simulink model "inverted_pendulum_2023b"  (R2023b)
settings: Solver=VariableStepAuto  StartTime=0.0  StopTime=double(Tsim)  RelTol=1e-3
InitFcn:
  | x0 = [0.0, 0, pi, 0.2];
  | measurementNoiseVariance = 1e-5 * [1, 1, 1, 1];
  | dt = 1e-3;
  | Tsim = 3;
settings Model: Creator=ka59symi  LastModifiedBy=ka59symi

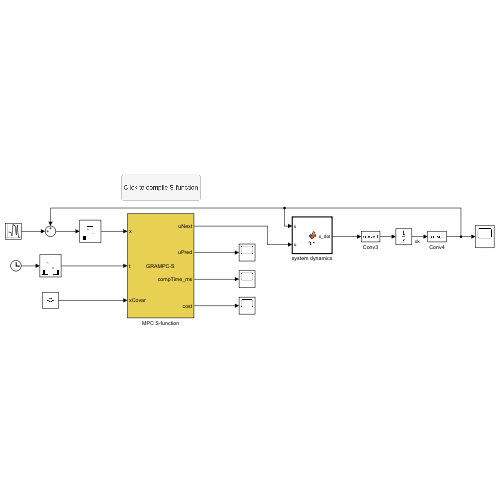
[thumbnail: Simulink's stored preview of the top-level diagram]
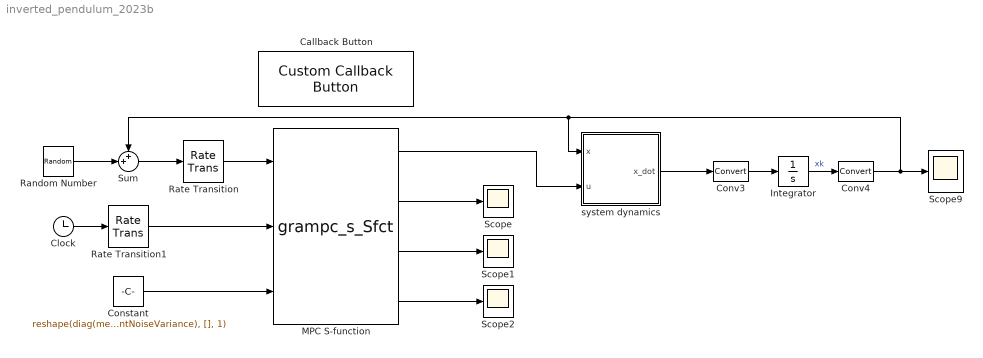
== system inverted_pendulum_2023b ==
  Callback Button : CustomCallbackButton  Configuration="{\"components\":[{\"name\":\"BackgroundImageComponent\",\"settings\":{\"image\":{\"size\":[0,0],\"src\":\"default\",\"srcOrientation\":\"Right\"},\"position\":[0,0,1,1]}},{\"name\":\"ButtonStateComponent\",\"settings\":{\"buttonType\":\"momentary\",\"clickFcn\":\"clc;\\nclear all;\\n\\npath_to_grampc = fileparts(fileparts(cd));\\n\\nprobfct_inc = fullfile(cd, 'inverted_pendulum_problem_description.hpp');\\nprobfct_src = fullfile(cd, 'inverted_pendulum_problem_description.cpp');\\ns_function  = fullfile(cd, 'grampc_s_Sfct.cpp');\\n\\naddpath(fullfile(path_to_grampc, 'matlab'));\\n\\nmake_Sfunction(path_to_grampc, probfct_inc, probfct_src, s_function);\",\"onValue\":1,\"position\":[0,0,1,1],\"pressDelay\":\"500\",\"pressFcn\":\"\",\"repeatInterval\":\"0\",\"states\":[{\"horizontalAlignment\":\"center\",\"image\":{\"position\":[0,0,1,1],\"size\":[1,1],\"src\":\"default\",\"srcOrientation\":\"Right\"},\"label\":{\"color\":[0.01176470588,0.01176470588,0.01176470588,1],\"icon\":{\"size\":[0,0],\"src\":\"default\",\"srcOrientation\":\"Right\"},\"iconPlacement\":\"left\",\"opacity\":1,\"show\":true,\"text\":{\"content\":\"Click to compile S-function\",\"font\":\"Helvetica\",\"fontSize\":15}},\"labelOffset\":[0,0],\"verticalAlignment\":\"middle\"},{\"horizontalAlignment\":\"center\",\"image\":{\"position\":[0,0,1,1],\"size\":[1,1],\"src\":\"default\",\"srcOrientation\":\"Right\"},\"label\":{\"color\":[0.01176470588,0.01176470588,0.01176470588,1],\"icon\":{\"size\":[0,0],\"src\":\"default\",\"srcOrientation\":\"Right\"},\"iconPlacement\":\"left\",\"opacity\":1,\"show\":true,\"text\":{\"content\":\"Click to compile S-function\",\"font\":\"Helvetica\",\"fontSize\":15}},\"labelOffset\":[0,0],\"verticalAlignment\":\"middle\"},{\"horizontalAlignment\":\"center\",\"image\":{\"position\":[0,0,1,1],\"size\":[1,1],\"src\":\"default\",\"srcOrientation\":\"Right\"},\"label\":{\"color\":[0.01176470588,0.01176470588,0.01176470588,1],\"icon\":{\"size\":[0,0],\"src\":\"default\",\"srcOrientation\":\"Right\"},\"iconPlacement\":\"left\",\"opacity\":1,\"show\":true,\"text\":{\"content\":\"Click to compile S-function\",\"font\":\"Helvetica\",\"fontSize\":15}},\"labelOffset\":[0,0],\"verticalAlignment\":\"middle\"},{\"horizontalAlignment\":\"center\",\"image\":{\"position\":[0,0,1,1],\"size\":[1,1],\"src\":\"default\",\"srcOrientation\":\"Right\"},\"label\":{\"color\":[0.01176470588,0.01176470588,0.01176470588,1],\"icon\":{\"size\":[0,0],\"src\":\"default\",\"srcOrientation\":\"Right\"},\"iconPlacement\":\"left\",\"opacity\":1,\"show\":true,\"text\":{\"content\":\"Click to compile S-function\",\"font\":\"Helvetica\",\"fontSize\":15}},\"labelOffset\":[0,0],\"verticalAlignment\":\"middle\"}]}},{\"name\":\"ForegroundImageComponent\",\"settings\":{\"image\":{\"size\":[0,0],\"src\":\"default\",\"srcOrientation\":\"Right\"},\"isForeground\":1,\"position\":[0,0,1,1]}}],\"settings\":{\"BindingType\":\"standalone\",\"backgroundColor\":[244,244,244,1],\"backgroundOffset\":0.2,\"backgroundOpacity\":1,\"fixedAspectRatio\":\"off\",\"foregroundColor\":[0.01176470588,0.01176470588,0.01176470588,1],\"migratedFromLegacy\":true,\"useBackgroundColor\":true,\"variant\":\"callback\",\"version\":\"R2023a\"},\"type\":\"Button\"}"  CustomBackgroundColor="{\"color\":[0.9568627451,0.9568627451,0.9568627451],\"show\":true}"
  Clock : Clock
  Constant : Constant  Value=reshape(diag(measurementNoiseVariance), [], 1)  VectorParams1D=off
  Conv3 : DataTypeConversion  SaturateOnIntegerOverflow=off  RndMeth=Floor
  Conv4 : DataTypeConversion  SaturateOnIntegerOverflow=off  RndMeth=Floor
  Integrator : Integrator  InitialCondition=x0
  MPC S-function : S-Function  FunctionName=grampc_s_Sfct  SFunctionDeploymentMode=off  EnableBusSupport=off
      mask Display:
      | port_label('input',1,'x')
      | port_label('input',2,'t')
      | port_label('input',3,'xCovar')
      | 
      | port_label('output',1,'uNext')
      | port_label('output',2,'uPred')
      | port_label('output',3,'compTime_ms')
      | port_label('output',4,'cost')
      | 
      | disp('GRAMPC-S')
  Random Number : RandomNumber  Mean=zeros(4,1)  Variance=measurementNoiseVariance  SampleTime=dt
  Rate Transition : RateTransition  OutPortSampleTime=dt
  Rate Transition1 : RateTransition  OutPortSampleTime=dt
  Scope{,1..2,9} (4 alike) : Scope
  Sum : Sum  Inputs=++|
  system dynamics : MATLAB Function  TreatAsAtomicUnit=on
  wires:
  Rate Transition/1 -> MPC S-function/1
  Random Number/1 -> Sum/2
  MPC S-function/3 -> Scope1/1
  MPC S-function/4 -> Scope2/1
  Sum/1 -> Rate Transition/1
  MPC S-function/2 -> Scope/1
  MPC S-function/1 -> system dynamics/2(u)
  Clock/1 -> Rate Transition1/1
  Integrator/1 -> Conv4/1  "xk"
  Constant/1 -> MPC S-function/3
  system dynamics/1(x_dot) -> Conv3/1
  Rate Transition1/1 -> MPC S-function/2
  Conv4/1 -> system dynamics/1(x), Sum/1, Scope9/1
  Conv3/1 -> Integrator/1

== matlab function inverted_pendulum_2023b/system dynamics ==
  data: x input; u input; x_dot output
function x_dot = fcn(x, u)
    x_dot = zeros(1, 4);

    x_dot(1) = x(2);
    x_dot(2) = u(1);
    x_dot(3) = x(4);
    x_dot(4) = -(2e-3*x(4)+0.2*(0.15*u(1)*cos(x(3))+0.15*9.81*sin(x(3))))/(1.3e-3+(0.2*0.2)*0.15);
end
